simulink model "basic_pid_position"  (R2015a)
settings: Solver=ode45  StartTime=0.0  StopTime=10.0  RelTol=1e-3
values from neighbouring files (symbols this model uses):
  K_d = 0.005    [parameters.m]
  K_i = 0.1    [parameters.m]
  K_p = 0.025    [parameters.m]
undefined symbols (not defined in the file or in its folder): pid
libraries: simulink x1, simulink_extras x1
settings Model: Creator=preston  LastModifiedBy=preston

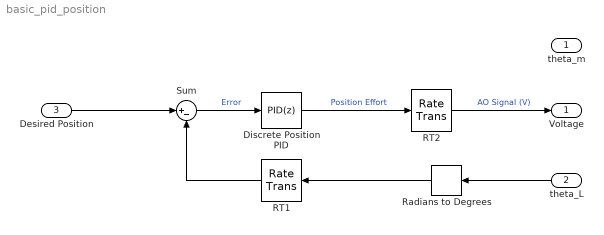
== system basic_pid_position ==
  theta_m : Inport
  theta_L : Inport  Port=2
  Desired Position : Inport  Port=3
  Discrete Position PID : simulink/Continuous/PID Controller  Controller=PID  TimeDomain=Discrete-time  SampleTime=-1  IntegratorMethod=Backward Euler  FilterMethod=Forward Euler  Form=Parallel  UseFilter=off  ControllerParametersSource=internal  P=K_p  I=K_i  D=K_d  N=pid.N  InitialConditionSource=internal  InitialConditionForIntegrator=0  InitialConditionForFilter=0  ExternalReset=none  LimitOutput=on  UpperSaturationLimit=2  LowerSaturationLimit=-2  LinearizeAsGain=off  AntiWindupMode=none  Kb=1  TrackingMode=off  Kt=1  PParamMin=[]  PParamMax=[]  IParamMin=[]  IParamMax=[]  DParamMin=[]  DParamMax=[]  NParamMin=[]  NParamMax=[]  KbParamMin=[]  KbParamMax=[]  KtParamMin=[]  KtParamMax=[]  POutMin=[]  POutMax=[]  IOutMin=[]  IOutMax=[]  DOutMin=[]  DOutMax=[]  NOutMin=[]  NOutMax=[]  KbOutMin=[]  KbOutMax=[]  KtOutMin=[]  KtOutMax=[]  IntegratorOutMin=[]  IntegratorOutMax=[]  FilterOutMin=[]  FilterOutMax=[]  SumOutMin=[]  SumOutMax=[]  SumI1OutMin=[]  SumI1OutMax=[]  SumI2OutMin=[]  SumI2OutMax=[]  SumI3OutMin=[]  SumI3OutMax=[]  SumDOutMin=[]  SumDOutMax=[]  SaturationOutMin=[]  SaturationOutMax=[]  IntegratorContinuousStateAttributes=''  IntegratorStateMustResolveToSignalObject=off  IntegratorRTWStateStorageClass=Auto  FilterContinuousStateAttributes=''  FilterStateMustResolveToSignalObject=off  FilterRTWStateStorageClass=Auto  DifferentiatorICPrevScaledInput=0  DifferentiatorOutMin=[]  DifferentiatorOutMax=[]
  RT1 : RateTransition  OutPortSampleTime=T_sample_control
  RT2 : RateTransition
  Radians to Degrees : simulink_extras/Transformations/Radians to Degrees
  Sum : Sum  Inputs=|+-
  Voltage : Outport
  wires:
  Discrete Position PID/1 -> RT2/1  "Position Effort"
  Sum/1 -> Discrete Position PID/1  "Error"
  RT1/1 -> Sum/2
  theta_L/1 -> Radians to Degrees/1
  RT2/1 -> Voltage/1  "AO Signal (V)"
  Radians to Degrees/1 -> RT1/1
  Desired Position/1 -> Sum/1
